simulink subsystem "AngularAccelerationSubsystem"  (R2023b)
settings: Solver=VariableStepAuto  StartTime=0.0  StopTime=10.0  RelTol=1e-3
settings Model: Creator=FRESH  LastModifiedBy=FRESH

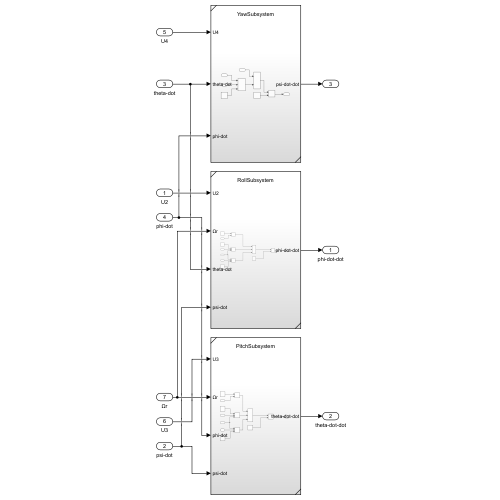
[thumbnail: Simulink's stored preview of the top-level diagram]
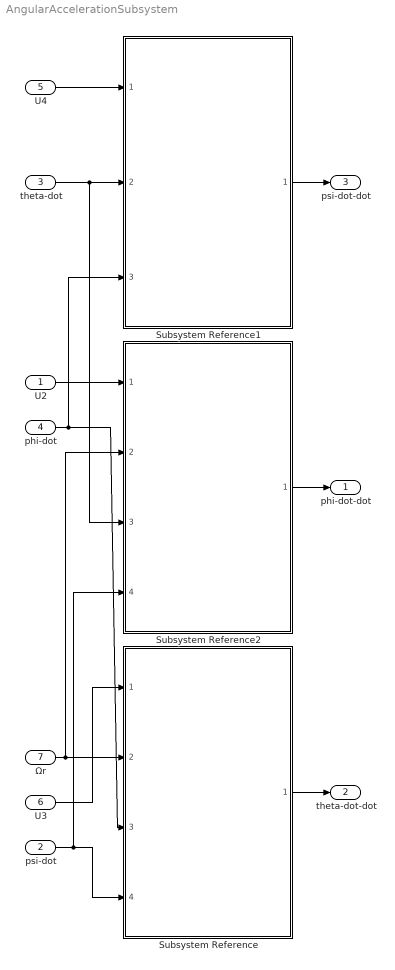
== system AngularAccelerationSubsystem ==
  U2 : Inport
  psi-dot : Inport  Port=2
  theta-dot : Inport  Port=3
  phi-dot : Inport  Port=4
  U4 : Inport  Port=5
  U3 : Inport  Port=6
  Ωr : Inport  Port=7
  Subsystem Reference : Subsystem  ReferencedSubsystem=PitchSubsystem
  Subsystem Reference1 : Subsystem  ReferencedSubsystem=YawSubsystem
  Subsystem Reference2 : Subsystem  ReferencedSubsystem=RollSubsystem
  phi-dot-dot : Outport
  theta-dot-dot : Outport  Port=2
  psi-dot-dot : Outport  Port=3
  wires:
  Subsystem Reference1/1 -> psi-dot-dot/1
  U4/1 -> Subsystem Reference1/1
  Ωr/1 -> Subsystem Reference/2, Subsystem Reference2/2
  theta-dot/1 -> Subsystem Reference1/2, Subsystem Reference2/3
  U2/1 -> Subsystem Reference2/1
  phi-dot/1 -> Subsystem Reference/3, Subsystem Reference1/3
  U3/1 -> Subsystem Reference/1
  psi-dot/1 -> Subsystem Reference/4, Subsystem Reference2/4
  Subsystem Reference2/1 -> phi-dot-dot/1
  Subsystem Reference/1 -> theta-dot-dot/1
